simulink model "test_mdl_NI"  (R2018a)
settings: Solver=VariableStepAuto  StartTime=0.0  StopTime=10.0  RelTol=1e-3
(part 10 of 24)

== system test_mdl_NI/Subsystem/GWM/OTAPhysGWM_ECGtoSODCMC_Ox1B9114D8 ==
  in_port : Inport
  OTAPhysGWM_ECGtoSODCMC : Terminator
  bus_selector : BusSelector  OutputSignals=OTAPhysGWM_ECGtoSODCMC
  wires:
  in_port/1 -> bus_selector/1  "OTAPhysGWM_ECGtoSODCMC_Ox1B9114D8"
  bus_selector/1 -> OTAPhysGWM_ECGtoSODCMC/1  "<OTAPhysGWM_ECGtoSODCMC>"

== system test_mdl_NI/Subsystem/GWM/OTAPhysGWM_ECGtoSODCMD_Ox1B9118D8 ==
  in_port : Inport
  OTAPhysGWM_ECGtoSODCMD : Terminator
  bus_selector : BusSelector  OutputSignals=OTAPhysGWM_ECGtoSODCMD
  wires:
  in_port/1 -> bus_selector/1  "OTAPhysGWM_ECGtoSODCMD_Ox1B9118D8"
  bus_selector/1 -> OTAPhysGWM_ECGtoSODCMD/1  "<OTAPhysGWM_ECGtoSODCMD>"

== system test_mdl_NI/Subsystem/GWM/OTAPhysGWM_ECGtoSODL_Ox1B9188D8 ==
  in_port : Inport
  OTAPhysGWM_ECGtoSODL : Terminator
  bus_selector : BusSelector  OutputSignals=OTAPhysGWM_ECGtoSODL
  wires:
  in_port/1 -> bus_selector/1  "OTAPhysGWM_ECGtoSODL_Ox1B9188D8"
  bus_selector/1 -> OTAPhysGWM_ECGtoSODL/1  "<OTAPhysGWM_ECGtoSODL>"

== system test_mdl_NI/Subsystem/GWM/OTAPhysGWM_ECGtoSODR_Ox1B918CD8 ==
  in_port : Inport
  OTAPhysGWM_ECGtoSODR : Terminator
  bus_selector : BusSelector  OutputSignals=OTAPhysGWM_ECGtoSODR
  wires:
  in_port/1 -> bus_selector/1  "OTAPhysGWM_ECGtoSODR_Ox1B918CD8"
  bus_selector/1 -> OTAPhysGWM_ECGtoSODR/1  "<OTAPhysGWM_ECGtoSODR>"

== system test_mdl_NI/Subsystem/GWM/OffBrdChrg_Signals2_Ox27F ==
  in_port : Inport
  OfbChrgClearAll_B_Rq : Terminator
  OfbChrgGoTDelete_B_Rq : Terminator
  OfbChrgGoTElement_D_Rq : Terminator
  OfbChrgGoTExtHtr_D_Rq : Terminator
  OfbChrgGoTHr_T_Rq : Terminator
  OfbChrgGoTMnte_D_Rq : Terminator
  OfbChrgGoTOn_D_Rq : Terminator
  OfbChrgGoTPrcond_D_Rq : Terminator
  OfbChrgGoTTouch_D_Rq : Terminator
  OfbChrgGoTUpdate_B_Rq : Terminator
  OfbChrgPrflUpdate_B_Rq : Terminator
  bus_selector : BusSelector  OutputSignals=OfbChrgClearAll_B_Rq,OfbChrgGoTDelete_B_Rq,OfbChrgGoTElement_D_Rq,OfbChrgGoTExtHtr_D_Rq,OfbChrgGoTHr_T_Rq,OfbChrgGoTMnte_D_Rq,OfbChrgGoTOn_D_Rq,OfbChrgGoTPrcond_D_Rq,OfbChrgGoTTouch_D_Rq,OfbChrgGoTUpdate_B_Rq,OfbChrgPrflUpdate_B_Rq
  wires:
  in_port/1 -> bus_selector/1  "OffBrdChrg_Signals2_Ox27F"
  bus_selector/1 -> OfbChrgClearAll_B_Rq/1  "<OfbChrgClearAll_B_Rq>"
  bus_selector/2 -> OfbChrgGoTDelete_B_Rq/1  "<OfbChrgGoTDelete_B_Rq>"
  bus_selector/3 -> OfbChrgGoTElement_D_Rq/1  "<OfbChrgGoTElement_D_Rq>"
  bus_selector/4 -> OfbChrgGoTExtHtr_D_Rq/1  "<OfbChrgGoTExtHtr_D_Rq>"
  bus_selector/5 -> OfbChrgGoTHr_T_Rq/1  "<OfbChrgGoTHr_T_Rq>"
  bus_selector/6 -> OfbChrgGoTMnte_D_Rq/1  "<OfbChrgGoTMnte_D_Rq>"
  bus_selector/7 -> OfbChrgGoTOn_D_Rq/1  "<OfbChrgGoTOn_D_Rq>"
  bus_selector/8 -> OfbChrgGoTPrcond_D_Rq/1  "<OfbChrgGoTPrcond_D_Rq>"
  bus_selector/9 -> OfbChrgGoTTouch_D_Rq/1  "<OfbChrgGoTTouch_D_Rq>"
  bus_selector/10 -> OfbChrgGoTUpdate_B_Rq/1  "<OfbChrgGoTUpdate_B_Rq>"
  bus_selector/11 -> OfbChrgPrflUpdate_B_Rq/1  "<OfbChrgPrflUpdate_B_Rq>"

== system test_mdl_NI/Subsystem/GWM/OffBrdChrg_Signals_Ox212 ==
  in_port : Inport
  OfbChrgLocIdTrgt_No_Rq : Terminator
  OfbChrgLocIdUns_B_Rq : Terminator
  OfbChrgPrflWkdy_No_Rq : Terminator
  OfbChrgPrflWknd_No_Rq : Terminator
  OfbChrgSetDelete_B_Rq : Terminator
  OfbChrgSetNow_D_Rq : Terminator
  OfbChrgToPcWkdy_D_Actl : Terminator
  OfbChrgToPcWknd_D_Actl : Terminator
  bus_selector : BusSelector  OutputSignals=OfbChrgLocIdTrgt_No_Rq,OfbChrgLocIdUns_B_Rq,OfbChrgPrflWkdy_No_Rq,OfbChrgPrflWknd_No_Rq,OfbChrgSetDelete_B_Rq,OfbChrgSetNow_D_Rq,OfbChrgToPcWkdy_D_Actl,OfbChrgToPcWknd_D_Actl
  wires:
  in_port/1 -> bus_selector/1  "OffBrdChrg_Signals_Ox212"
  bus_selector/1 -> OfbChrgLocIdTrgt_No_Rq/1  "<OfbChrgLocIdTrgt_No_Rq>"
  bus_selector/2 -> OfbChrgLocIdUns_B_Rq/1  "<OfbChrgLocIdUns_B_Rq>"
  bus_selector/3 -> OfbChrgPrflWkdy_No_Rq/1  "<OfbChrgPrflWkdy_No_Rq>"
  bus_selector/4 -> OfbChrgPrflWknd_No_Rq/1  "<OfbChrgPrflWknd_No_Rq>"
  bus_selector/5 -> OfbChrgSetDelete_B_Rq/1  "<OfbChrgSetDelete_B_Rq>"
  bus_selector/6 -> OfbChrgSetNow_D_Rq/1  "<OfbChrgSetNow_D_Rq>"
  bus_selector/7 -> OfbChrgToPcWkdy_D_Actl/1  "<OfbChrgToPcWkdy_D_Actl>"
  bus_selector/8 -> OfbChrgToPcWknd_D_Actl/1  "<OfbChrgToPcWknd_D_Actl>"

== system test_mdl_NI/Subsystem/GWM/PARSEDFuncGWM_ECG_FD1_Ox1BAFFCD8 ==
  in_port : Inport
  PARSEDFuncGWM_ECG : Terminator
  bus_selector : BusSelector  OutputSignals=PARSEDFuncGWM_ECG
  wires:
  in_port/1 -> bus_selector/1  "PARSEDFuncGWM_ECG_FD1_Ox1BAFFCD8"
  bus_selector/1 -> PARSEDFuncGWM_ECG/1  "<PARSEDFuncGWM_ECG>"

== system test_mdl_NI/Subsystem/GWM/PARSEDPhysGWM_ECGtoABS_Ox1BA0A0D8 ==
  in_port : Inport
  PARSEDPhysGWM_ECGtoABS : Terminator
  bus_selector : BusSelector  OutputSignals=PARSEDPhysGWM_ECGtoABS
  wires:
  in_port/1 -> bus_selector/1  "PARSEDPhysGWM_ECGtoABS_Ox1BA0A0D8"
  bus_selector/1 -> PARSEDPhysGWM_ECGtoABS/1  "<PARSEDPhysGWM_ECGtoABS>"

== system test_mdl_NI/Subsystem/GWM/PARSEDPhysGWM_ECGtoCCM_Ox1BA054D8 ==
  in_port : Inport
  PARSEDPhysGWM_ECGtoCCM : Terminator
  bus_selector : BusSelector  OutputSignals=PARSEDPhysGWM_ECGtoCCM
  wires:
  in_port/1 -> bus_selector/1  "PARSEDPhysGWM_ECGtoCCM_Ox1BA054D8"
  bus_selector/1 -> PARSEDPhysGWM_ECGtoCCM/1  "<PARSEDPhysGWM_ECGtoCCM>"

== system test_mdl_NI/Subsystem/GWM/PARSEDPhysGWM_ECGtoIPMA_Ox1BA084D8 ==
  in_port : Inport
  PARSEDPhysGWM_ECGtoIPMA : Terminator
  bus_selector : BusSelector  OutputSignals=PARSEDPhysGWM_ECGtoIPMA
  wires:
  in_port/1 -> bus_selector/1  "PARSEDPhysGWM_ECGtoIPMA_Ox1BA084D8"
  bus_selector/1 -> PARSEDPhysGWM_ECGtoIPMA/1  "<PARSEDPhysGWM_ECGtoIPMA>"

== system test_mdl_NI/Subsystem/GWM/PARSEDPhysGWM_ECGtoPCM_Ox1BA040D8 ==
  in_port : Inport
  PARSEDPhysGWM_ECGtoPCM : Terminator
  bus_selector : BusSelector  OutputSignals=PARSEDPhysGWM_ECGtoPCM
  wires:
  in_port/1 -> bus_selector/1  "PARSEDPhysGWM_ECGtoPCM_Ox1BA040D8"
  bus_selector/1 -> PARSEDPhysGWM_ECGtoPCM/1  "<PARSEDPhysGWM_ECGtoPCM>"

== system test_mdl_NI/Subsystem/GWM/PARSEDPhysGWM_ECGtoSODCMC_Ox1BA114D8 ==
  in_port : Inport
  PARSEDPhysGWM_ECGtoSODCMC : Terminator
  bus_selector : BusSelector  OutputSignals=PARSEDPhysGWM_ECGtoSODCMC
  wires:
  in_port/1 -> bus_selector/1  "PARSEDPhysGWM_ECGtoSODCMC_Ox1BA114D8"
  bus_selector/1 -> PARSEDPhysGWM_ECGtoSODCMC/1  "<PARSEDPhysGWM_ECGtoSODCMC>"

== system test_mdl_NI/Subsystem/GWM/PARSEDPhysGWM_ECGtoSODCMD_Ox1BA118D8 ==
  in_port : Inport
  PARSEDPhysGWM_ECGtoSODCMD : Terminator
  bus_selector : BusSelector  OutputSignals=PARSEDPhysGWM_ECGtoSODCMD
  wires:
  in_port/1 -> bus_selector/1  "PARSEDPhysGWM_ECGtoSODCMD_Ox1BA118D8"
  bus_selector/1 -> PARSEDPhysGWM_ECGtoSODCMD/1  "<PARSEDPhysGWM_ECGtoSODCMD>"

== system test_mdl_NI/Subsystem/GWM/PARSEDPhysGWM_ECGtoSODL_Ox1BA188D8 ==
  in_port : Inport
  PARSEDPhysGWM_ECGtoSODL : Terminator
  bus_selector : BusSelector  OutputSignals=PARSEDPhysGWM_ECGtoSODL
  wires:
  in_port/1 -> bus_selector/1  "PARSEDPhysGWM_ECGtoSODL_Ox1BA188D8"
  bus_selector/1 -> PARSEDPhysGWM_ECGtoSODL/1  "<PARSEDPhysGWM_ECGtoSODL>"

== system test_mdl_NI/Subsystem/GWM/PARSEDPhysGWM_ECGtoSODR_Ox1BA18CD8 ==
  in_port : Inport
  PARSEDPhysGWM_ECGtoSODR : Terminator
  bus_selector : BusSelector  OutputSignals=PARSEDPhysGWM_ECGtoSODR
  wires:
  in_port/1 -> bus_selector/1  "PARSEDPhysGWM_ECGtoSODR_Ox1BA18CD8"
  bus_selector/1 -> PARSEDPhysGWM_ECGtoSODR/1  "<PARSEDPhysGWM_ECGtoSODR>"

== system test_mdl_NI/Subsystem/GWM/PARSEDPhysGWMtoSOBDMC_FD1_Ox1BA044D8 ==
  in_port : Inport
  PARSEDPhysGWM_ECGtoHPCM : Terminator
  bus_selector : BusSelector  OutputSignals=PARSEDPhysGWM_ECGtoHPCM
  wires:
  in_port/1 -> bus_selector/1  "PARSEDPhysGWMtoSOBDMC_FD1_Ox1BA044D8"
  bus_selector/1 -> PARSEDPhysGWM_ECGtoHPCM/1  "<PARSEDPhysGWM_ECGtoHPCM>"

== system test_mdl_NI/Subsystem/GWM/PARSEDPushFcGWM_ECGtoABS_Ox1BB0A0D8 ==
  in_port : Inport
  PARSEDPhysGWM_ECG2toABS : Terminator
  bus_selector : BusSelector  OutputSignals=PARSEDPhysGWM_ECG2toABS
  wires:
  in_port/1 -> bus_selector/1  "PARSEDPushFcGWM_ECGtoABS_Ox1BB0A0D8"
  bus_selector/1 -> PARSEDPhysGWM_ECG2toABS/1  "<PARSEDPhysGWM_ECG2toABS>"

== system test_mdl_NI/Subsystem/GWM/PARSEDPushFcGWM_ECGtoPCM_Ox1BB040D8 ==
  in_port : Inport
  PARSEDPhysGWM_ECG2toPCM : Terminator
  bus_selector : BusSelector  OutputSignals=PARSEDPhysGWM_ECG2toPCM
  wires:
  in_port/1 -> bus_selector/1  "PARSEDPushFcGWM_ECGtoPCM_Ox1BB040D8"
  bus_selector/1 -> PARSEDPhysGWM_ECG2toPCM/1  "<PARSEDPhysGWM_ECG2toPCM>"

== system test_mdl_NI/Subsystem/GWM/PHEV_Battery_Data1_FD1_Ox2E4 ==
  in_port : Inport
  BattAuxCnnct_B_Cmd : Terminator
  bus_selector : BusSelector  OutputSignals=BattAuxCnnct_B_Cmd
  wires:
  in_port/1 -> bus_selector/1  "PHEV_Battery_Data1_FD1_Ox2E4"
  bus_selector/1 -> BattAuxCnnct_B_Cmd/1  "<BattAuxCnnct_B_Cmd>"

== system test_mdl_NI/Subsystem/GWM/ParkAid_Aud_Warn_CmdM_FD1_Ox30A ==
  in_port : Inport
  Cta_D_Rq : Terminator
  PrkAidAcsyFront_D_RqDrv : Terminator
  PrkAidAcsyRear_D_RqDrv : Terminator
  PrkAidFront_D_RqDrv : Terminator
  PrkAidRear_D_RqDrv : Terminator
  Sod_D_Rq : Terminator
  SteEffort_D_Rq : Terminator
  bus_selector : BusSelector  OutputSignals=Cta_D_Rq,PrkAidAcsyFront_D_RqDrv,PrkAidAcsyRear_D_RqDrv,PrkAidFront_D_RqDrv,PrkAidRear_D_RqDrv,Sod_D_Rq,SteEffort_D_Rq
  wires:
  in_port/1 -> bus_selector/1  "ParkAid_Aud_Warn_CmdM_FD1_Ox30A"
  bus_selector/1 -> Cta_D_Rq/1  "<Cta_D_Rq>"
  bus_selector/2 -> PrkAidAcsyFront_D_RqDrv/1  "<PrkAidAcsyFront_D_RqDrv>"
  bus_selector/3 -> PrkAidAcsyRear_D_RqDrv/1  "<PrkAidAcsyRear_D_RqDrv>"
  bus_selector/4 -> PrkAidFront_D_RqDrv/1  "<PrkAidFront_D_RqDrv>"
  bus_selector/5 -> PrkAidRear_D_RqDrv/1  "<PrkAidRear_D_RqDrv>"
  bus_selector/6 -> Sod_D_Rq/1  "<Sod_D_Rq>"
  bus_selector/7 -> SteEffort_D_Rq/1  "<SteEffort_D_Rq>"

== system test_mdl_NI/Subsystem/GWM/Pass_Dr_Stat_FD1_Ox333 ==
  in_port : Inport
  BLISLEDStatPassSide : Terminator
  ChildLckFdbckRp_B_Stat : Terminator
  Memory_1_SwPsngr_Stat : Terminator
  Memory_2_SwPsngr_Stat : Terminator
  Memory_3_SwPsngr_Stat : Terminator
  Pasngr_Lock_Sw_Cnt : Terminator
  Pasngr_Lock_Sw_Stat : Terminator
  RollCode_No_ActlPdm : Terminator
  WndwPsngrSide_D_Stat : Terminator
  bus_selector : BusSelector  OutputSignals=BLISLEDStatPassSide,ChildLckFdbckRp_B_Stat,Memory_1_SwPsngr_Stat,Memory_2_SwPsngr_Stat,Memory_3_SwPsngr_Stat,Pasngr_Lock_Sw_Cnt,Pasngr_Lock_Sw_Stat,RollCode_No_ActlPdm,WndwPsngrSide_D_Stat
  wires:
  in_port/1 -> bus_selector/1  "Pass_Dr_Stat_FD1_Ox333"
  bus_selector/1 -> BLISLEDStatPassSide/1  "<BLISLEDStatPassSide>"
  bus_selector/2 -> ChildLckFdbckRp_B_Stat/1  "<ChildLckFdbckRp_B_Stat>"
  bus_selector/3 -> Memory_1_SwPsngr_Stat/1  "<Memory_1_SwPsngr_Stat>"
  bus_selector/4 -> Memory_2_SwPsngr_Stat/1  "<Memory_2_SwPsngr_Stat>"
  bus_selector/5 -> Memory_3_SwPsngr_Stat/1  "<Memory_3_SwPsngr_Stat>"
  bus_selector/6 -> Pasngr_Lock_Sw_Cnt/1  "<Pasngr_Lock_Sw_Cnt>"
  bus_selector/7 -> Pasngr_Lock_Sw_Stat/1  "<Pasngr_Lock_Sw_Stat>"
  bus_selector/8 -> RollCode_No_ActlPdm/1  "<RollCode_No_ActlPdm>"
  bus_selector/9 -> WndwPsngrSide_D_Stat/1  "<WndwPsngrSide_D_Stat>"

== system test_mdl_NI/Subsystem/GWM/Personality_APIM_Data_FD1_Ox3E2 ==
  in_port : Inport
  CtrStkDsplyOp_D_Rq : Terminator
  CtrStkFeatConfigActl : Terminator
  CtrStkFeatNoActl : Terminator
  CtrStkPersIndex_D_Actl : Terminator
  Pers1OptIn_B_Stats : Terminator
  Pers2OptIn_B_Stats : Terminator
  Pers3OptIn_B_Stats : Terminator
  Pers4OptIn_B_Stats : Terminator
  PersStore_D_Rq : Terminator
  bus_selector : BusSelector  OutputSignals=CtrStkDsplyOp_D_Rq,CtrStkFeatConfigActl,CtrStkFeatNoActl,CtrStkPersIndex_D_Actl,Pers1OptIn_B_Stats,Pers2OptIn_B_Stats,Pers3OptIn_B_Stats,Pers4OptIn_B_Stats,PersStore_D_Rq
  wires:
  in_port/1 -> bus_selector/1  "Personality_APIM_Data_FD1_Ox3E2"
  bus_selector/1 -> CtrStkDsplyOp_D_Rq/1  "<CtrStkDsplyOp_D_Rq>"
  bus_selector/2 -> CtrStkFeatConfigActl/1  "<CtrStkFeatConfigActl>"
  bus_selector/3 -> CtrStkFeatNoActl/1  "<CtrStkFeatNoActl>"
  bus_selector/4 -> CtrStkPersIndex_D_Actl/1  "<CtrStkPersIndex_D_Actl>"
  bus_selector/5 -> Pers1OptIn_B_Stats/1  "<Pers1OptIn_B_Stats>"
  bus_selector/6 -> Pers2OptIn_B_Stats/1  "<Pers2OptIn_B_Stats>"
  bus_selector/7 -> Pers3OptIn_B_Stats/1  "<Pers3OptIn_B_Stats>"
  bus_selector/8 -> Pers4OptIn_B_Stats/1  "<Pers4OptIn_B_Stats>"
  bus_selector/9 -> PersStore_D_Rq/1  "<PersStore_D_Rq>"

== system test_mdl_NI/Subsystem/GWM/Personality_BCM2_Data_FD1_Ox3EB ==
  in_port : Inport
  AssocConfirm_D_Actl : Terminator
  EmPrflKeyAssoc_D_Stat : Terminator
  EmPrflNo_D_Stat : Terminator
  Pers1Key_D_Stat : Terminator
  Pers2Key_D_Stat : Terminator
  Pers3Key_D_Stat : Terminator
  Pers4Key_D_Stat : Terminator
  PersConflict_D_Actl : Terminator
  PersNoPos_D_Actl : Terminator
  PersNo_D_Actl : Terminator
  PersRecallSrc_D_Actl : Terminator
  PersSetupAccessCtrl : Terminator
  PersSetupRestr_D_Actl : Terminator
  PersSetup_No_Actl : Terminator
  RecallEvent_No_Cnt : Terminator
  VehKeyActv_D_Stat : Terminator
  bus_selector : BusSelector  OutputSignals=AssocConfirm_D_Actl,EmPrflKeyAssoc_D_Stat,EmPrflNo_D_Stat,Pers1Key_D_Stat,Pers2Key_D_Stat,Pers3Key_D_Stat,Pers4Key_D_Stat,PersConflict_D_Actl,PersNoPos_D_Actl,PersNo_D_Actl,PersRecallSrc_D_Actl,PersSetupAccessCtrl,PersSetupRestr_D_Actl,PersSetup_No_Actl,RecallEvent_No_Cnt,VehKeyActv_D_Stat
  wires:
  in_port/1 -> bus_selector/1  "Personality_BCM2_Data_FD1_Ox3EB"
  bus_selector/1 -> AssocConfirm_D_Actl/1  "<AssocConfirm_D_Actl>"
  bus_selector/2 -> EmPrflKeyAssoc_D_Stat/1  "<EmPrflKeyAssoc_D_Stat>"
  bus_selector/3 -> EmPrflNo_D_Stat/1  "<EmPrflNo_D_Stat>"
  bus_selector/4 -> Pers1Key_D_Stat/1  "<Pers1Key_D_Stat>"
  bus_selector/5 -> Pers2Key_D_Stat/1  "<Pers2Key_D_Stat>"
  bus_selector/6 -> Pers3Key_D_Stat/1  "<Pers3Key_D_Stat>"
  bus_selector/7 -> Pers4Key_D_Stat/1  "<Pers4Key_D_Stat>"
  bus_selector/8 -> PersConflict_D_Actl/1  "<PersConflict_D_Actl>"
  bus_selector/9 -> PersNoPos_D_Actl/1  "<PersNoPos_D_Actl>"
  bus_selector/10 -> PersNo_D_Actl/1  "<PersNo_D_Actl>"
  bus_selector/11 -> PersRecallSrc_D_Actl/1  "<PersRecallSrc_D_Actl>"
  bus_selector/12 -> PersSetupAccessCtrl/1  "<PersSetupAccessCtrl>"
  bus_selector/13 -> PersSetupRestr_D_Actl/1  "<PersSetupRestr_D_Actl>"
  bus_selector/14 -> PersSetup_No_Actl/1  "<PersSetup_No_Actl>"
  bus_selector/15 -> RecallEvent_No_Cnt/1  "<RecallEvent_No_Cnt>"
  bus_selector/16 -> VehKeyActv_D_Stat/1  "<VehKeyActv_D_Stat>"

== system test_mdl_NI/Subsystem/GWM/Personality_Data_FD1_Ox3E0 ==
  in_port : Inport
  MsgCntrDsplyOp_D_Rq : Terminator
  MsgCntrFeatConfigRq : Terminator
  MsgCntrFeatNoRq : Terminator
  MsgCntrPersIndex_D_Rq : Terminator
  bus_selector : BusSelector  OutputSignals=MsgCntrDsplyOp_D_Rq,MsgCntrFeatConfigRq,MsgCntrFeatNoRq,MsgCntrPersIndex_D_Rq
  wires:
  in_port/1 -> bus_selector/1  "Personality_Data_FD1_Ox3E0"
  bus_selector/1 -> MsgCntrDsplyOp_D_Rq/1  "<MsgCntrDsplyOp_D_Rq>"
  bus_selector/2 -> MsgCntrFeatConfigRq/1  "<MsgCntrFeatConfigRq>"
  bus_selector/3 -> MsgCntrFeatNoRq/1  "<MsgCntrFeatNoRq>"
  bus_selector/4 -> MsgCntrPersIndex_D_Rq/1  "<MsgCntrPersIndex_D_Rq>"

== system test_mdl_NI/Subsystem/GWM/PowerDistData_2_FD1_Ox36A ==
  in_port : Inport
  AirCondCluBatt_D_Falt : Terminator
  AirCondCluGnd_D_Falt : Terminator
  AirCondCluLife_D_Falt : Terminator
  AirCondCluOpen_D_Falt : Terminator
  AirCondClu_D_Stat : Terminator
  BattChlrLifeLim_D_Falt : Terminator
  BattChlrOpnCirct_D_Falt : Terminator
  BattChlrShrtBatt_D_Falt : Terminator
  BattChlrShrtGrnd_D_Falt : Terminator
  BattTracLifeLim_D_Falt : Terminator
  BattTracLow_D_Falt : Terminator
  BattTracOpnCirct_D_Falt : Terminator
  BattTracShrtBatt_D_Falt : Terminator
  BattTracShrtGrnd_D_Falt : Terminator
  bus_selector : BusSelector  OutputSignals=AirCondCluBatt_D_Falt,AirCondCluGnd_D_Falt,AirCondCluLife_D_Falt,AirCondCluOpen_D_Falt,AirCondClu_D_Stat,BattChlrLifeLim_D_Falt,BattChlrOpnCirct_D_Falt,BattChlrShrtBatt_D_Falt,BattChlrShrtGrnd_D_Falt,BattTracLifeLim_D_Falt,BattTracLow_D_Falt,BattTracOpnCirct_D_Falt,BattTracShrtBatt_D_Falt,BattTracShrtGrnd_D_Falt
  wires:
  in_port/1 -> bus_selector/1  "PowerDistData_2_FD1_Ox36A"
  bus_selector/1 -> AirCondCluBatt_D_Falt/1  "<AirCondCluBatt_D_Falt>"
  bus_selector/2 -> AirCondCluGnd_D_Falt/1  "<AirCondCluGnd_D_Falt>"
  bus_selector/3 -> AirCondCluLife_D_Falt/1  "<AirCondCluLife_D_Falt>"
  bus_selector/4 -> AirCondCluOpen_D_Falt/1  "<AirCondCluOpen_D_Falt>"
  bus_selector/5 -> AirCondClu_D_Stat/1  "<AirCondClu_D_Stat>"
  bus_selector/6 -> BattChlrLifeLim_D_Falt/1  "<BattChlrLifeLim_D_Falt>"
  bus_selector/7 -> BattChlrOpnCirct_D_Falt/1  "<BattChlrOpnCirct_D_Falt>"
  bus_selector/8 -> BattChlrShrtBatt_D_Falt/1  "<BattChlrShrtBatt_D_Falt>"
  bus_selector/9 -> BattChlrShrtGrnd_D_Falt/1  "<BattChlrShrtGrnd_D_Falt>"
  bus_selector/10 -> BattTracLifeLim_D_Falt/1  "<BattTracLifeLim_D_Falt>"
  bus_selector/11 -> BattTracLow_D_Falt/1  "<BattTracLow_D_Falt>"
  bus_selector/12 -> BattTracOpnCirct_D_Falt/1  "<BattTracOpnCirct_D_Falt>"
  bus_selector/13 -> BattTracShrtBatt_D_Falt/1  "<BattTracShrtBatt_D_Falt>"
  bus_selector/14 -> BattTracShrtGrnd_D_Falt/1  "<BattTracShrtGrnd_D_Falt>"

== system test_mdl_NI/Subsystem/GWM/PowerDist_Data1_FD1_Ox390 ==
  in_port : Inport
  BattChlrSov_D_Stat : Terminator
  BattTracClntVlv_D_Stat : Terminator
  CabnEvapSovFront_D_Stat : Terminator
  bus_selector : BusSelector  OutputSignals=BattChlrSov_D_Stat,BattTracClntVlv_D_Stat,CabnEvapSovFront_D_Stat
  wires:
  in_port/1 -> bus_selector/1  "PowerDist_Data1_FD1_Ox390"
  bus_selector/1 -> BattChlrSov_D_Stat/1  "<BattChlrSov_D_Stat>"
  bus_selector/2 -> BattTracClntVlv_D_Stat/1  "<BattTracClntVlv_D_Stat>"
  bus_selector/3 -> CabnEvapSovFront_D_Stat/1  "<CabnEvapSovFront_D_Stat>"

== system test_mdl_NI/Subsystem/GWM/Power_Liftgate_Stat_FD1_Ox313 ==
  in_port : Inport
  DrLckCnt_No_ActlTgate : Terminator
  DrTGate_D_Rq : Terminator
  DrTgateChime2_D_Rq : Terminator
  Power_Liftgate_Mode_Stt : Terminator
  PwLftgtIntSw_B_Stat : Terminator
  bus_selector : BusSelector  OutputSignals=DrLckCnt_No_ActlTgate,DrTGate_D_Rq,DrTgateChime2_D_Rq,Power_Liftgate_Mode_Stt,PwLftgtIntSw_B_Stat
  wires:
  in_port/1 -> bus_selector/1  "Power_Liftgate_Stat_FD1_Ox313"
  bus_selector/1 -> DrLckCnt_No_ActlTgate/1  "<DrLckCnt_No_ActlTgate>"
  bus_selector/2 -> DrTGate_D_Rq/1  "<DrTGate_D_Rq>"
  bus_selector/3 -> DrTgateChime2_D_Rq/1  "<DrTgateChime2_D_Rq>"
  bus_selector/4 -> Power_Liftgate_Mode_Stt/1  "<Power_Liftgate_Mode_Stt>"
  bus_selector/5 -> PwLftgtIntSw_B_Stat/1  "<PwLftgtIntSw_B_Stat>"

== system test_mdl_NI/Subsystem/GWM/RCMSerialNumber_FD1_Ox454 ==
  in_port : Inport
  RCMSerialNoByte{1..8} (8 alike) : Terminator
  bus_selector : BusSelector  OutputSignals=RCMSerialNoByte1,RCMSerialNoByte2,RCMSerialNoByte3,RCMSerialNoByte4,RCMSerialNoByte5,RCMSerialNoByte6,RCMSerialNoByte7,RCMSerialNoByte8
  wires:
  in_port/1 -> bus_selector/1  "RCMSerialNumber_FD1_Ox454"
  bus_selector/1 -> RCMSerialNoByte1/1  "<RCMSerialNoByte1>"
  bus_selector/2 -> RCMSerialNoByte2/1  "<RCMSerialNoByte2>"
  bus_selector/3 -> RCMSerialNoByte3/1  "<RCMSerialNoByte3>"
  bus_selector/4 -> RCMSerialNoByte4/1  "<RCMSerialNoByte4>"
  bus_selector/5 -> RCMSerialNoByte5/1  "<RCMSerialNoByte5>"
  bus_selector/6 -> RCMSerialNoByte6/1  "<RCMSerialNoByte6>"
  bus_selector/7 -> RCMSerialNoByte7/1  "<RCMSerialNoByte7>"
  bus_selector/8 -> RCMSerialNoByte8/1  "<RCMSerialNoByte8>"

== system test_mdl_NI/Subsystem/GWM/RCMStatusMessage2_FD1_Ox4C ==
  in_port : Inport
  EDRTriggerEvntSync : Terminator
  FirstRowBuckleDriver : Terminator
  FirstRowBuckleMid : Terminator
  FirstRowBucklePsngr : Terminator
  PassRstrnInd_Req : Terminator
  PsngrFrntDetct_D_Actl : Terminator
  RILReq : Terminator
  RstrnImpactEvntStatus : Terminator
  SecondRowBuckleDriver : Terminator
  SecondRowBuckleMid : Terminator
  SecondRowBucklePsngr : Terminator
  bus_selector : BusSelector  OutputSignals=EDRTriggerEvntSync,FirstRowBuckleDriver,FirstRowBuckleMid,FirstRowBucklePsngr,PassRstrnInd_Req,PsngrFrntDetct_D_Actl,RILReq,RstrnImpactEvntStatus,SecondRowBuckleDriver,SecondRowBuckleMid,SecondRowBucklePsngr
  wires:
  in_port/1 -> bus_selector/1  "RCMStatusMessage2_FD1_Ox4C"
  bus_selector/1 -> EDRTriggerEvntSync/1  "<EDRTriggerEvntSync>"
  bus_selector/2 -> FirstRowBuckleDriver/1  "<FirstRowBuckleDriver>"
  bus_selector/3 -> FirstRowBuckleMid/1  "<FirstRowBuckleMid>"
  bus_selector/4 -> FirstRowBucklePsngr/1  "<FirstRowBucklePsngr>"
  bus_selector/5 -> PassRstrnInd_Req/1  "<PassRstrnInd_Req>"
  bus_selector/6 -> PsngrFrntDetct_D_Actl/1  "<PsngrFrntDetct_D_Actl>"
  bus_selector/7 -> RILReq/1  "<RILReq>"
  bus_selector/8 -> RstrnImpactEvntStatus/1  "<RstrnImpactEvntStatus>"
  bus_selector/9 -> SecondRowBuckleDriver/1  "<SecondRowBuckleDriver>"
  bus_selector/10 -> SecondRowBuckleMid/1  "<SecondRowBuckleMid>"
  bus_selector/11 -> SecondRowBucklePsngr/1  "<SecondRowBucklePsngr>"

== system test_mdl_NI/Subsystem/GWM/SmartChargingData_ECG_1_Ox306 ==
  in_port : Inport
  ScLocDelete_B_RqCld : Terminator
  ScLocId_No_RqCld : Terminator
  ScLocLattDeg_An_RqCld : Terminator
  ScLocLattFrct_An_RqCld : Terminator
  ScLocLattPostv_B_RqCld : Terminator
  ScLocLongDeg_An_RqCld : Terminator
  ScLocLongFrct_An_RqCld : Terminator
  ScLocLongPostv_B_RqCld : Terminator
  bus_selector : BusSelector  OutputSignals=ScLocDelete_B_RqCld,ScLocId_No_RqCld,ScLocLattDeg_An_RqCld,ScLocLattFrct_An_RqCld,ScLocLattPostv_B_RqCld,ScLocLongDeg_An_RqCld,ScLocLongFrct_An_RqCld,ScLocLongPostv_B_RqCld
  wires:
  in_port/1 -> bus_selector/1  "SmartChargingData_ECG_1_Ox306"
  bus_selector/1 -> ScLocDelete_B_RqCld/1  "<ScLocDelete_B_RqCld>"
  bus_selector/2 -> ScLocId_No_RqCld/1  "<ScLocId_No_RqCld>"
  bus_selector/3 -> ScLocLattDeg_An_RqCld/1  "<ScLocLattDeg_An_RqCld>"
  bus_selector/4 -> ScLocLattFrct_An_RqCld/1  "<ScLocLattFrct_An_RqCld>"
  bus_selector/5 -> ScLocLattPostv_B_RqCld/1  "<ScLocLattPostv_B_RqCld>"
  bus_selector/6 -> ScLocLongDeg_An_RqCld/1  "<ScLocLongDeg_An_RqCld>"
  bus_selector/7 -> ScLocLongFrct_An_RqCld/1  "<ScLocLongFrct_An_RqCld>"
  bus_selector/8 -> ScLocLongPostv_B_RqCld/1  "<ScLocLongPostv_B_RqCld>"

== system test_mdl_NI/Subsystem/GWM/SmartChargingData_ECG_2_Ox307 ==
  in_port : Inport
  ScChrgDurSet_D_RqCld : Terminator
  ScChrgDur_T_RqCld : Terminator
  ScChrgPrfl_No_RqCld : Terminator
  ScChrgToPc_Pc_RqCld : Terminator
  ScDayOfWeekId_D_RqCld : Terminator
  ScLocRdius_L_RqCld : Terminator
  ScLocSetId_No_RqCld : Terminator
  bus_selector : BusSelector  OutputSignals=ScChrgDurSet_D_RqCld,ScChrgDur_T_RqCld,ScChrgPrfl_No_RqCld,ScChrgToPc_Pc_RqCld,ScDayOfWeekId_D_RqCld,ScLocRdius_L_RqCld,ScLocSetId_No_RqCld
  wires:
  in_port/1 -> bus_selector/1  "SmartChargingData_ECG_2_Ox307"
  bus_selector/1 -> ScChrgDurSet_D_RqCld/1  "<ScChrgDurSet_D_RqCld>"
  bus_selector/2 -> ScChrgDur_T_RqCld/1  "<ScChrgDur_T_RqCld>"
  bus_selector/3 -> ScChrgPrfl_No_RqCld/1  "<ScChrgPrfl_No_RqCld>"
  bus_selector/4 -> ScChrgToPc_Pc_RqCld/1  "<ScChrgToPc_Pc_RqCld>"
  bus_selector/5 -> ScDayOfWeekId_D_RqCld/1  "<ScDayOfWeekId_D_RqCld>"
  bus_selector/6 -> ScLocRdius_L_RqCld/1  "<ScLocRdius_L_RqCld>"
  bus_selector/7 -> ScLocSetId_No_RqCld/1  "<ScLocSetId_No_RqCld>"

== system test_mdl_NI/Subsystem/GWM/SmartChargingData_ECG_3_Ox308 ==
  in_port : Inport
  AirAmb_Te_ActlCld : Terminator
  ChrgToPcEdit_Pc_RqCld : Terminator
  GoTEditHr_T_RqCld : Terminator
  GoTEditMnte_T_RqCld : Terminator
  PrcondEdit_D_RqCld : Terminator
  ScChrgrPwMax_Pw_RqCld : Terminator
  ScEnbl_D_RqCld : Terminator
  ScFreshDataEnbl_B_Rq : Terminator
  ScLocPwId_No_RqCld : Terminator
  ScMnSoc_Pc_RqCld : Terminator
  bus_selector : BusSelector  OutputSignals=AirAmb_Te_ActlCld,ChrgToPcEdit_Pc_RqCld,GoTEditHr_T_RqCld,GoTEditMnte_T_RqCld,PrcondEdit_D_RqCld,ScChrgrPwMax_Pw_RqCld,ScEnbl_D_RqCld,ScFreshDataEnbl_B_Rq,ScLocPwId_No_RqCld,ScMnSoc_Pc_RqCld
  wires:
  in_port/1 -> bus_selector/1  "SmartChargingData_ECG_3_Ox308"
  bus_selector/1 -> AirAmb_Te_ActlCld/1  "<AirAmb_Te_ActlCld>"
  bus_selector/2 -> ChrgToPcEdit_Pc_RqCld/1  "<ChrgToPcEdit_Pc_RqCld>"
  bus_selector/3 -> GoTEditHr_T_RqCld/1  "<GoTEditHr_T_RqCld>"
  bus_selector/4 -> GoTEditMnte_T_RqCld/1  "<GoTEditMnte_T_RqCld>"
  bus_selector/5 -> PrcondEdit_D_RqCld/1  "<PrcondEdit_D_RqCld>"
  bus_selector/6 -> ScChrgrPwMax_Pw_RqCld/1  "<ScChrgrPwMax_Pw_RqCld>"
  bus_selector/7 -> ScEnbl_D_RqCld/1  "<ScEnbl_D_RqCld>"
  bus_selector/8 -> ScFreshDataEnbl_B_Rq/1  "<ScFreshDataEnbl_B_Rq>"
  bus_selector/9 -> ScLocPwId_No_RqCld/1  "<ScLocPwId_No_RqCld>"
  bus_selector/10 -> ScMnSoc_Pc_RqCld/1  "<ScMnSoc_Pc_RqCld>"

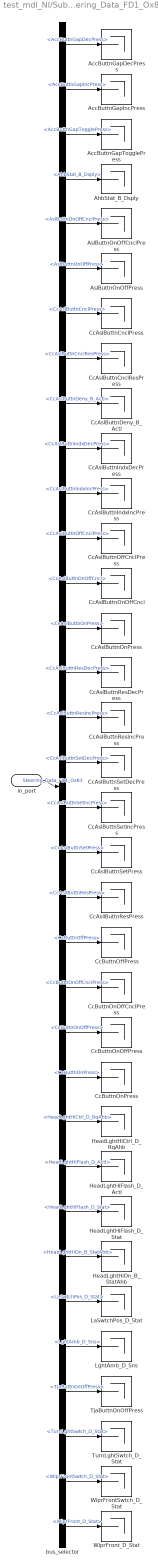
== system test_mdl_NI/Subsystem/GWM/Steering_Data_FD1_Ox83 ==
  in_port : Inport
  AccButtnGapDecPress : Terminator
  AccButtnGapIncPress : Terminator
  AccButtnGapTogglePress : Terminator
  AhbStat_B_Dsply : Terminator
  AslButtnOnOffCnclPress : Terminator
  AslButtnOnOffPress : Terminator
  CcAslButtnCnclPress : Terminator
  CcAslButtnCnclResPress : Terminator
  CcAslButtnDeny_B_Actl : Terminator
  CcAslButtnIndxDecPress : Terminator
  CcAslButtnIndxIncPress : Terminator
  CcAslButtnOffCnclPress : Terminator
  CcAslButtnOnOffCncl : Terminator
  CcAslButtnOnPress : Terminator
  CcAslButtnResDecPress : Terminator
  CcAslButtnResIncPress : Terminator
  CcAslButtnSetDecPress : Terminator
  CcAslButtnSetIncPress : Terminator
  CcAslButtnSetPress : Terminator
  CcAsllButtnResPress : Terminator
  CcButtnOffPress : Terminator
  CcButtnOnOffCnclPress : Terminator
  CcButtnOnOffPress : Terminator
  CcButtnOnPress : Terminator
  HeadLghtHiCtrl_D_RqAhb : Terminator
  HeadLghtHiFlash_D_Actl : Terminator
  HeadLghtHiFlash_D_Stat : Terminator
  HeadLghtHiOn_B_StatAhb : Terminator
  LaSwtchPos_D_Stat : Terminator
  LghtAmb_D_Sns : Terminator
  TjaButtnOnOffPress : Terminator
  TurnLghtSwtch_D_Stat : Terminator
  WiprFrontSwtch_D_Stat : Terminator
  WiprFront_D_Stat : Terminator
  bus_selector : BusSelector  OutputSignals=AccButtnGapDecPress,AccButtnGapIncPress,AccButtnGapTogglePress,AhbStat_B_Dsply,AslButtnOnOffCnclPress,AslButtnOnOffPress,CcAslButtnCnclPress,CcAslButtnCnclResPress,CcAslButtnDeny_B_Actl,CcAslButtnIndxDecPress,CcAslButtnIndxIncPress,CcAslButtnOffCnclPress,CcAslButtnOnOffCncl,CcAslButtnOnPress,CcAslButtnResDecPress,CcAslButtnResIncPress,CcAslButtnSetDecPress,CcAslButtnSetIncPress,CcAslButtnSetPress,CcAsllButtnResPress,CcButtnOffPress,CcButtnOnOffCnclPress,CcButtnOnOffPress,CcButtnOnPress,HeadLghtHiCtrl_D_RqAhb,HeadLghtHiFlash_D_Actl,HeadLghtHiFlash_D_Stat,HeadLghtHiOn_B_StatAhb,LaSwtchPos_D_Stat,LghtAmb_D_Sns,TjaButtnOnOffPress,TurnLghtSwtch_D_Stat,WiprFrontSwtch_D_Stat,WiprFront_D_Stat
  wires:
  in_port/1 -> bus_selector/1  "Steering_Data_FD1_Ox83"
  bus_selector/1 -> AccButtnGapDecPress/1  "<AccButtnGapDecPress>"
  bus_selector/2 -> AccButtnGapIncPress/1  "<AccButtnGapIncPress>"
  bus_selector/3 -> AccButtnGapTogglePress/1  "<AccButtnGapTogglePress>"
  bus_selector/4 -> AhbStat_B_Dsply/1  "<AhbStat_B_Dsply>"
  bus_selector/5 -> AslButtnOnOffCnclPress/1  "<AslButtnOnOffCnclPress>"
  bus_selector/6 -> AslButtnOnOffPress/1  "<AslButtnOnOffPress>"
  bus_selector/7 -> CcAslButtnCnclPress/1  "<CcAslButtnCnclPress>"
  bus_selector/8 -> CcAslButtnCnclResPress/1  "<CcAslButtnCnclResPress>"
  bus_selector/9 -> CcAslButtnDeny_B_Actl/1  "<CcAslButtnDeny_B_Actl>"
  bus_selector/10 -> CcAslButtnIndxDecPress/1  "<CcAslButtnIndxDecPress>"
  bus_selector/11 -> CcAslButtnIndxIncPress/1  "<CcAslButtnIndxIncPress>"
  bus_selector/12 -> CcAslButtnOffCnclPress/1  "<CcAslButtnOffCnclPress>"
  bus_selector/13 -> CcAslButtnOnOffCncl/1  "<CcAslButtnOnOffCncl>"
  bus_selector/14 -> CcAslButtnOnPress/1  "<CcAslButtnOnPress>"
  bus_selector/15 -> CcAslButtnResDecPress/1  "<CcAslButtnResDecPress>"
  bus_selector/16 -> CcAslButtnResIncPress/1  "<CcAslButtnResIncPress>"
  bus_selector/17 -> CcAslButtnSetDecPress/1  "<CcAslButtnSetDecPress>"
  bus_selector/18 -> CcAslButtnSetIncPress/1  "<CcAslButtnSetIncPress>"
  bus_selector/19 -> CcAslButtnSetPress/1  "<CcAslButtnSetPress>"
  bus_selector/20 -> CcAsllButtnResPress/1  "<CcAsllButtnResPress>"
  bus_selector/21 -> CcButtnOffPress/1  "<CcButtnOffPress>"
  bus_selector/22 -> CcButtnOnOffCnclPress/1  "<CcButtnOnOffCnclPress>"
  bus_selector/23 -> CcButtnOnOffPress/1  "<CcButtnOnOffPress>"
  bus_selector/24 -> CcButtnOnPress/1  "<CcButtnOnPress>"
  bus_selector/25 -> HeadLghtHiCtrl_D_RqAhb/1  "<HeadLghtHiCtrl_D_RqAhb>"
  bus_selector/26 -> HeadLghtHiFlash_D_Actl/1  "<HeadLghtHiFlash_D_Actl>"
  bus_selector/27 -> HeadLghtHiFlash_D_Stat/1  "<HeadLghtHiFlash_D_Stat>"
  bus_selector/28 -> HeadLghtHiOn_B_StatAhb/1  "<HeadLghtHiOn_B_StatAhb>"
  bus_selector/29 -> LaSwtchPos_D_Stat/1  "<LaSwtchPos_D_Stat>"
  bus_selector/30 -> LghtAmb_D_Sns/1  "<LghtAmb_D_Sns>"
  bus_selector/31 -> TjaButtnOnOffPress/1  "<TjaButtnOnOffPress>"
  bus_selector/32 -> TurnLghtSwtch_D_Stat/1  "<TurnLghtSwtch_D_Stat>"
  bus_selector/33 -> WiprFrontSwtch_D_Stat/1  "<WiprFrontSwtch_D_Stat>"
  bus_selector/34 -> WiprFront_D_Stat/1  "<WiprFront_D_Stat>"

== system test_mdl_NI/Subsystem/GWM/Steering_Wheel_Data2_FD1_Ox81 ==
  in_port : Inport
  SelDrvMdeDec_B_RqDrv : Terminator
  SelDrvMdeInc_B_RqDrv : Terminator
  SelDrvMdeSwtch_D_Stat4 : Terminator
  SteEffortInc_B_RqDrv : Terminator
  SteWhlSwtchBack_B_Stat : Terminator
  SteWhlSwtchDown_B_Stat : Terminator
  SteWhlSwtchHome_B_Stat : Terminator
  SteWhlSwtchHud_B_Stat : Terminator
  SteWhlSwtchInfo_B_Stat : Terminator
  SteWhlSwtchIod_B_Stat : Terminator
  SteWhlSwtchLeft_B_Stat : Terminator
  SteWhlSwtchMed_B_Stat : Terminator
  SteWhlSwtchMenu_B_Stat : Terminator
  SteWhlSwtchNav_B_Stat : Terminator
  SteWhlSwtchOk_B_Stat : Terminator
  SteWhlSwtchPhon_B_Stat : Terminator
  SteWhlSwtchRght_B_Stat : Terminator
  SteWhlSwtchSet_B_Stat : Terminator
  SteWhlSwtchUp_B_Stat : Terminator
  SteWhlSwtchView_B_Stat : Terminator
  SuspDampInc_B_RqDrv : Terminator
  bus_selector : BusSelector  OutputSignals=SelDrvMdeDec_B_RqDrv,SelDrvMdeInc_B_RqDrv,SelDrvMdeSwtch_D_Stat4,SteEffortInc_B_RqDrv,SteWhlSwtchBack_B_Stat,SteWhlSwtchDown_B_Stat,SteWhlSwtchHome_B_Stat,SteWhlSwtchHud_B_Stat,SteWhlSwtchInfo_B_Stat,SteWhlSwtchIod_B_Stat,SteWhlSwtchLeft_B_Stat,SteWhlSwtchMed_B_Stat,SteWhlSwtchMenu_B_Stat,SteWhlSwtchNav_B_Stat,SteWhlSwtchOk_B_Stat,SteWhlSwtchPhon_B_Stat,SteWhlSwtchRght_B_Stat,SteWhlSwtchSet_B_Stat,SteWhlSwtchUp_B_Stat,SteWhlSwtchView_B_Stat,SuspDampInc_B_RqDrv
  wires:
  in_port/1 -> bus_selector/1  "Steering_Wheel_Data2_FD1_Ox81"
  bus_selector/1 -> SelDrvMdeDec_B_RqDrv/1  "<SelDrvMdeDec_B_RqDrv>"
  bus_selector/2 -> SelDrvMdeInc_B_RqDrv/1  "<SelDrvMdeInc_B_RqDrv>"
  bus_selector/3 -> SelDrvMdeSwtch_D_Stat4/1  "<SelDrvMdeSwtch_D_Stat4>"
  bus_selector/4 -> SteEffortInc_B_RqDrv/1  "<SteEffortInc_B_RqDrv>"
  bus_selector/5 -> SteWhlSwtchBack_B_Stat/1  "<SteWhlSwtchBack_B_Stat>"
  bus_selector/6 -> SteWhlSwtchDown_B_Stat/1  "<SteWhlSwtchDown_B_Stat>"
  bus_selector/7 -> SteWhlSwtchHome_B_Stat/1  "<SteWhlSwtchHome_B_Stat>"
  bus_selector/8 -> SteWhlSwtchHud_B_Stat/1  "<SteWhlSwtchHud_B_Stat>"
  bus_selector/9 -> SteWhlSwtchInfo_B_Stat/1  "<SteWhlSwtchInfo_B_Stat>"
  bus_selector/10 -> SteWhlSwtchIod_B_Stat/1  "<SteWhlSwtchIod_B_Stat>"
  bus_selector/11 -> SteWhlSwtchLeft_B_Stat/1  "<SteWhlSwtchLeft_B_Stat>"
  bus_selector/12 -> SteWhlSwtchMed_B_Stat/1  "<SteWhlSwtchMed_B_Stat>"
  bus_selector/13 -> SteWhlSwtchMenu_B_Stat/1  "<SteWhlSwtchMenu_B_Stat>"
  bus_selector/14 -> SteWhlSwtchNav_B_Stat/1  "<SteWhlSwtchNav_B_Stat>"
  bus_selector/15 -> SteWhlSwtchOk_B_Stat/1  "<SteWhlSwtchOk_B_Stat>"
  bus_selector/16 -> SteWhlSwtchPhon_B_Stat/1  "<SteWhlSwtchPhon_B_Stat>"
  bus_selector/17 -> SteWhlSwtchRght_B_Stat/1  "<SteWhlSwtchRght_B_Stat>"
  bus_selector/18 -> SteWhlSwtchSet_B_Stat/1  "<SteWhlSwtchSet_B_Stat>"
  bus_selector/19 -> SteWhlSwtchUp_B_Stat/1  "<SteWhlSwtchUp_B_Stat>"
  bus_selector/20 -> SteWhlSwtchView_B_Stat/1  "<SteWhlSwtchView_B_Stat>"
  bus_selector/21 -> SuspDampInc_B_RqDrv/1  "<SuspDampInc_B_RqDrv>"

== system test_mdl_NI/Subsystem/GWM/TCU_Send_Signals_FD1_Ox28B ==
  in_port : Inport
  EmgcyCallMute_D_Stat : Terminator
  OfbChrgSetSync_D_Rq : Terminator
  TelematicsSrvc_D_St : Terminator
  bus_selector : BusSelector  OutputSignals=EmgcyCallMute_D_Stat,OfbChrgSetSync_D_Rq,TelematicsSrvc_D_St
  wires:
  in_port/1 -> bus_selector/1  "TCU_Send_Signals_FD1_Ox28B"
  bus_selector/1 -> EmgcyCallMute_D_Stat/1  "<EmgcyCallMute_D_Stat>"
  bus_selector/2 -> OfbChrgSetSync_D_Rq/1  "<OfbChrgSetSync_D_Rq>"
  bus_selector/3 -> TelematicsSrvc_D_St/1  "<TelematicsSrvc_D_St>"

== system test_mdl_NI/Subsystem/GWM/TesterPhysicalReqVDM_FD1_Ox721 ==
  in_port : Inport
  TesterPhysicalReqVDM : Terminator
  bus_selector : BusSelector  OutputSignals=TesterPhysicalReqVDM
  wires:
  in_port/1 -> bus_selector/1  "TesterPhysicalReqVDM_FD1_Ox721"
  bus_selector/1 -> TesterPhysicalReqVDM/1  "<TesterPhysicalReqVDM>"

== system test_mdl_NI/Subsystem/GWM/TesterPhysicalResGWM_FD1_Ox71E ==
  in_port : Inport
  TesterPhysicalResGWM_F1 : Terminator
  bus_selector : BusSelector  OutputSignals=TesterPhysicalResGWM_F1
  wires:
  in_port/1 -> bus_selector/1  "TesterPhysicalResGWM_FD1_Ox71E"
  bus_selector/1 -> TesterPhysicalResGWM_F1/1  "<TesterPhysicalResGWM_F1>"

== system test_mdl_NI/Subsystem/GWM/Tire_Pressure_Data_FD1_Ox3B5 ==
  in_port : Inport
  Tire_Press_LF_Data : Terminator
  Tire_Press_LR_OLR_Data : Terminator
  Tire_Press_RF_Data : Terminator
  Tire_Press_RR_ORR_Data : Terminator
  bus_selector : BusSelector  OutputSignals=Tire_Press_LF_Data,Tire_Press_LR_OLR_Data,Tire_Press_RF_Data,Tire_Press_RR_ORR_Data
  wires:
  in_port/1 -> bus_selector/1  "Tire_Pressure_Data_FD1_Ox3B5"
  bus_selector/1 -> Tire_Press_LF_Data/1  "<Tire_Press_LF_Data>"
  bus_selector/2 -> Tire_Press_LR_OLR_Data/1  "<Tire_Press_LR_OLR_Data>"
  bus_selector/3 -> Tire_Press_RF_Data/1  "<Tire_Press_RF_Data>"
  bus_selector/4 -> Tire_Press_RR_ORR_Data/1  "<Tire_Press_RR_ORR_Data>"

== system test_mdl_NI/Subsystem/GWM/TrailerAid_Data3_FD1_Ox45C ==
  in_port : Inport
  TrlrAidEnbl_D2_Rq : Terminator
  TrlrAidSetup_D2_Rq : Terminator
  TrlrAnOffstDir_D_Mem : Terminator
  TrlrAnOffst_An_Mem : Terminator
  TrlrAxleToBmpr_L_Actl : Terminator
  TrlrBallToBmpr_L_Actl : Terminator
  TrlrIdType_D_Stat : Terminator
  TrlrId_No_Actl : Terminator
  TrlrRvrseCancl_B_Rq : Terminator
  TrlrTrgtOffst_L_Actl : Terminator
  TrlrTrgtPtrnId_No_Mem : Terminator
  TrlrTrgtToBmpr_L_Actl : Terminator
  bus_selector : BusSelector  OutputSignals=TrlrAidEnbl_D2_Rq,TrlrAidSetup_D2_Rq,TrlrAnOffstDir_D_Mem,TrlrAnOffst_An_Mem,TrlrAxleToBmpr_L_Actl,TrlrBallToBmpr_L_Actl,TrlrIdType_D_Stat,TrlrId_No_Actl,TrlrRvrseCancl_B_Rq,TrlrTrgtOffst_L_Actl,TrlrTrgtPtrnId_No_Mem,TrlrTrgtToBmpr_L_Actl
  wires:
  in_port/1 -> bus_selector/1  "TrailerAid_Data3_FD1_Ox45C"
  bus_selector/1 -> TrlrAidEnbl_D2_Rq/1  "<TrlrAidEnbl_D2_Rq>"
  bus_selector/2 -> TrlrAidSetup_D2_Rq/1  "<TrlrAidSetup_D2_Rq>"
  bus_selector/3 -> TrlrAnOffstDir_D_Mem/1  "<TrlrAnOffstDir_D_Mem>"
  bus_selector/4 -> TrlrAnOffst_An_Mem/1  "<TrlrAnOffst_An_Mem>"
  bus_selector/5 -> TrlrAxleToBmpr_L_Actl/1  "<TrlrAxleToBmpr_L_Actl>"
  bus_selector/6 -> TrlrBallToBmpr_L_Actl/1  "<TrlrBallToBmpr_L_Actl>"
  bus_selector/7 -> TrlrIdType_D_Stat/1  "<TrlrIdType_D_Stat>"
  bus_selector/8 -> TrlrId_No_Actl/1  "<TrlrId_No_Actl>"
  bus_selector/9 -> TrlrRvrseCancl_B_Rq/1  "<TrlrRvrseCancl_B_Rq>"
  bus_selector/10 -> TrlrTrgtOffst_L_Actl/1  "<TrlrTrgtOffst_L_Actl>"
  bus_selector/11 -> TrlrTrgtPtrnId_No_Mem/1  "<TrlrTrgtPtrnId_No_Mem>"
  bus_selector/12 -> TrlrTrgtToBmpr_L_Actl/1  "<TrlrTrgtToBmpr_L_Actl>"

== system test_mdl_NI/Subsystem/GWM/TrailerAid_Data_FD1_Ox45A ==
  in_port : Inport
  TrailCtlSwtch_B_Stat2 : Terminator
  TrlBrkInitOut_D_Rq : Terminator
  bus_selector : BusSelector  OutputSignals=TrailCtlSwtch_B_Stat2,TrlBrkInitOut_D_Rq
  wires:
  in_port/1 -> bus_selector/1  "TrailerAid_Data_FD1_Ox45A"
  bus_selector/1 -> TrailCtlSwtch_B_Stat2/1  "<TrailCtlSwtch_B_Stat2>"
  bus_selector/2 -> TrlBrkInitOut_D_Rq/1  "<TrlBrkInitOut_D_Rq>"

== system test_mdl_NI/Subsystem/GWM/TrailerAid_Stat1_FD1_Ox452 ==
  in_port : Inport
  TrlrSnsId_No_Actl : Terminator
  bus_selector : BusSelector  OutputSignals=TrlrSnsId_No_Actl
  wires:
  in_port/1 -> bus_selector/1  "TrailerAid_Stat1_FD1_Ox452"
  bus_selector/1 -> TrlrSnsId_No_Actl/1  "<TrlrSnsId_No_Actl>"

== system test_mdl_NI/Subsystem/GWM/TrailerAid_Stat2_FD1_Ox457 ==
  in_port : Inport
  TrlrHitYaw_AnRate_Actl : Terminator
  TrlrHitchYaw_An_Actl : Terminator
  TrlrHitchYaw_D_Stat : Terminator
  TrlrYawWActl_D_Qf : Terminator
  TrlrYaw_W_Actl : Terminator
  bus_selector : BusSelector  OutputSignals=TrlrHitYaw_AnRate_Actl,TrlrHitchYaw_An_Actl,TrlrHitchYaw_D_Stat,TrlrYawWActl_D_Qf,TrlrYaw_W_Actl
  wires:
  in_port/1 -> bus_selector/1  "TrailerAid_Stat2_FD1_Ox457"
  bus_selector/1 -> TrlrHitYaw_AnRate_Actl/1  "<TrlrHitYaw_AnRate_Actl>"
  bus_selector/2 -> TrlrHitchYaw_An_Actl/1  "<TrlrHitchYaw_An_Actl>"
  bus_selector/3 -> TrlrHitchYaw_D_Stat/1  "<TrlrHitchYaw_D_Stat>"
  bus_selector/4 -> TrlrYawWActl_D_Qf/1  "<TrlrYawWActl_D_Qf>"
  bus_selector/5 -> TrlrYaw_W_Actl/1  "<TrlrYaw_W_Actl>"

== system test_mdl_NI/Subsystem/GWM/TrailerBrakeInfo_FD1_Ox445 ==
  in_port : Inport
  StopLamp_B_RqTrlrBrk : Terminator
  TrlBrkInitOut_D_Stat : Terminator
  TrlrBrkActCirct_B_Falt : Terminator
  TrlrBrkActCnnct_B_Actl : Terminator
  TrlrBrkCtl_B_Falt : Terminator
  TrlrBrkDcnnt_B_Actl : Terminator
  TrlrBrkDsply_B_Rq : Terminator
  TrlrBrkGain_No_Actl : Terminator
  TrlrBrkMde_D_Actl : Terminator
  TrlrBrkOut_No_Dsply : Terminator
  bus_selector : BusSelector  OutputSignals=StopLamp_B_RqTrlrBrk,TrlBrkInitOut_D_Stat,TrlrBrkActCirct_B_Falt,TrlrBrkActCnnct_B_Actl,TrlrBrkCtl_B_Falt,TrlrBrkDcnnt_B_Actl,TrlrBrkDsply_B_Rq,TrlrBrkGain_No_Actl,TrlrBrkMde_D_Actl,TrlrBrkOut_No_Dsply
  wires:
  in_port/1 -> bus_selector/1  "TrailerBrakeInfo_FD1_Ox445"
  bus_selector/1 -> StopLamp_B_RqTrlrBrk/1  "<StopLamp_B_RqTrlrBrk>"
  bus_selector/2 -> TrlBrkInitOut_D_Stat/1  "<TrlBrkInitOut_D_Stat>"
  bus_selector/3 -> TrlrBrkActCirct_B_Falt/1  "<TrlrBrkActCirct_B_Falt>"
  bus_selector/4 -> TrlrBrkActCnnct_B_Actl/1  "<TrlrBrkActCnnct_B_Actl>"
  bus_selector/5 -> TrlrBrkCtl_B_Falt/1  "<TrlrBrkCtl_B_Falt>"
  bus_selector/6 -> TrlrBrkDcnnt_B_Actl/1  "<TrlrBrkDcnnt_B_Actl>"
  bus_selector/7 -> TrlrBrkDsply_B_Rq/1  "<TrlrBrkDsply_B_Rq>"
  bus_selector/8 -> TrlrBrkGain_No_Actl/1  "<TrlrBrkGain_No_Actl>"
  bus_selector/9 -> TrlrBrkMde_D_Actl/1  "<TrlrBrkMde_D_Actl>"
  bus_selector/10 -> TrlrBrkOut_No_Dsply/1  "<TrlrBrkOut_No_Dsply>"

== system test_mdl_NI/Subsystem/GWM/TrailerInfo_2_FD1_Ox47A ==
  in_port : Inport
  TrlrAidCtl_U_RqDrv : Terminator
  TrlrAidSwtch_D_RqDrv : Terminator
  bus_selector : BusSelector  OutputSignals=TrlrAidCtl_U_RqDrv,TrlrAidSwtch_D_RqDrv
  wires:
  in_port/1 -> bus_selector/1  "TrailerInfo_2_FD1_Ox47A"
  bus_selector/1 -> TrlrAidCtl_U_RqDrv/1  "<TrlrAidCtl_U_RqDrv>"
  bus_selector/2 -> TrlrAidSwtch_D_RqDrv/1  "<TrlrAidSwtch_D_RqDrv>"

== system test_mdl_NI/Subsystem/GWM/TrailerInfo_FD1_Ox443 ==
  in_port : Inport
  ParkLampTrlrOut_B_Stat : Terminator
  StopLampTrlrOut_B_Stat : Terminator
  TrlrBattChrg_D_Stat : Terminator
  TrlrLampCnnct_B_Actl : Terminator
  TrlrLampCtl_D_Stat : Terminator
  TurnLampTrlrRl_B_Stat : Terminator
  TurnLampTrlrRr_B_Stat : Terminator
  bus_selector : BusSelector  OutputSignals=ParkLampTrlrOut_B_Stat,StopLampTrlrOut_B_Stat,TrlrBattChrg_D_Stat,TrlrLampCnnct_B_Actl,TrlrLampCtl_D_Stat,TurnLampTrlrRl_B_Stat,TurnLampTrlrRr_B_Stat
  wires:
  in_port/1 -> bus_selector/1  "TrailerInfo_FD1_Ox443"
  bus_selector/1 -> ParkLampTrlrOut_B_Stat/1  "<ParkLampTrlrOut_B_Stat>"
  bus_selector/2 -> StopLampTrlrOut_B_Stat/1  "<StopLampTrlrOut_B_Stat>"
  bus_selector/3 -> TrlrBattChrg_D_Stat/1  "<TrlrBattChrg_D_Stat>"
  bus_selector/4 -> TrlrLampCnnct_B_Actl/1  "<TrlrLampCnnct_B_Actl>"
  bus_selector/5 -> TrlrLampCtl_D_Stat/1  "<TrlrLampCtl_D_Stat>"
  bus_selector/6 -> TurnLampTrlrRl_B_Stat/1  "<TurnLampTrlrRl_B_Stat>"
  bus_selector/7 -> TurnLampTrlrRr_B_Stat/1  "<TurnLampTrlrRr_B_Stat>"

== system test_mdl_NI/Subsystem/GWM/Voltage_Power_Data2_FD1_Ox45F ==
  in_port : Inport
  CoolFanDcdc_D_Rq : Terminator
  DcdcClntFlw_D_Rq : Terminator
  bus_selector : BusSelector  OutputSignals=CoolFanDcdc_D_Rq,DcdcClntFlw_D_Rq
  wires:
  in_port/1 -> bus_selector/1  "Voltage_Power_Data2_FD1_Ox45F"
  bus_selector/1 -> CoolFanDcdc_D_Rq/1  "<CoolFanDcdc_D_Rq>"
  bus_selector/2 -> DcdcClntFlw_D_Rq/1  "<DcdcClntFlw_D_Rq>"

== system test_mdl_NI/Subsystem/GWM/Yaw_Data_FD1_Ox91 ==
  in_port : Inport
  VehRolWActl_D_Qf : Terminator
  VehRol_W_Actl : Terminator
  VehRollYawW_No_Cs : Terminator
  VehRollYaw_No_Cnt : Terminator
  VehYawWActl_D_Qf : Terminator
  VehYaw_W_Actl : Terminator
  bus_selector : BusSelector  OutputSignals=VehRolWActl_D_Qf,VehRol_W_Actl,VehRollYawW_No_Cs,VehRollYaw_No_Cnt,VehYawWActl_D_Qf,VehYaw_W_Actl
  wires:
  in_port/1 -> bus_selector/1  "Yaw_Data_FD1_Ox91"
  bus_selector/1 -> VehRolWActl_D_Qf/1  "<VehRolWActl_D_Qf>"
  bus_selector/2 -> VehRol_W_Actl/1  "<VehRol_W_Actl>"
  bus_selector/3 -> VehRollYawW_No_Cs/1  "<VehRollYawW_No_Cs>"
  bus_selector/4 -> VehRollYaw_No_Cnt/1  "<VehRollYaw_No_Cnt>"
  bus_selector/5 -> VehYawWActl_D_Qf/1  "<VehYawWActl_D_Qf>"
  bus_selector/6 -> VehYaw_W_Actl/1  "<VehYaw_W_Actl>"

== system test_mdl_NI/Subsystem/IPMA_ADAS/ACCDATA_2_Ox187 ==
  in_port : Inport
  CmbbBaSens_D_Rq : Terminator
  CmbbBrkDecel_A_Rq : Terminator
  CmbbBrkDecel_B_Rq : Terminator
  CmbbBrkDecel_No_Cnt : Terminator
  CmbbBrkDecel_No_Cs : Terminator
  CmbbBrkPrchg_D_Rq : Terminator
  HudBlk1_B_Rq : Terminator
  HudBlk2_B_Rq : Terminator
  HudBlk3_B_Rq : Terminator
  HudDsplyIntns_No_Actl : Terminator
  HudFlashRate_D_Actl : Terminator
  bus_selector : BusSelector  OutputSignals=CmbbBaSens_D_Rq,CmbbBrkDecel_A_Rq,CmbbBrkDecel_B_Rq,CmbbBrkDecel_No_Cnt,CmbbBrkDecel_No_Cs,CmbbBrkPrchg_D_Rq,HudBlk1_B_Rq,HudBlk2_B_Rq,HudBlk3_B_Rq,HudDsplyIntns_No_Actl,HudFlashRate_D_Actl
  wires:
  in_port/1 -> bus_selector/1  "ACCDATA_2_Ox187"
  bus_selector/1 -> CmbbBaSens_D_Rq/1  "<CmbbBaSens_D_Rq>"
  bus_selector/2 -> CmbbBrkDecel_A_Rq/1  "<CmbbBrkDecel_A_Rq>"
  bus_selector/3 -> CmbbBrkDecel_B_Rq/1  "<CmbbBrkDecel_B_Rq>"
  bus_selector/4 -> CmbbBrkDecel_No_Cnt/1  "<CmbbBrkDecel_No_Cnt>"
  bus_selector/5 -> CmbbBrkDecel_No_Cs/1  "<CmbbBrkDecel_No_Cs>"
  bus_selector/6 -> CmbbBrkPrchg_D_Rq/1  "<CmbbBrkPrchg_D_Rq>"
  bus_selector/7 -> HudBlk1_B_Rq/1  "<HudBlk1_B_Rq>"
  bus_selector/8 -> HudBlk2_B_Rq/1  "<HudBlk2_B_Rq>"
  bus_selector/9 -> HudBlk3_B_Rq/1  "<HudBlk3_B_Rq>"
  bus_selector/10 -> HudDsplyIntns_No_Actl/1  "<HudDsplyIntns_No_Actl>"
  bus_selector/11 -> HudFlashRate_D_Actl/1  "<HudFlashRate_D_Actl>"

== system test_mdl_NI/Subsystem/IPMA_ADAS/ACCDATA_3_Ox18A ==
  in_port : Inport
  AccFllwMde_B_Dsply : Terminator
  AccMemEnbl_B_RqDrv : Terminator
  AccMsgTxt_D2_Rq : Terminator
  AccStopMde_B_Dsply : Terminator
  AccStopRes_B_Dsply : Terminator
  AccStopStat_D_Dsply : Terminator
  AccTGap_B_Dsply : Terminator
  AccTGap_D_Dsply : Terminator
  AccTrgDist2_D_Dsply : Terminator
  AccWarn_D_Dsply : Terminator
  CadsAlignIncplt_B_Actl : Terminator
  CadsRadrBlck_B_Actl : Terminator
  CmbbPostEvnt_B_Dsply : Terminator
  FcwAudioWarn_B_Rq : Terminator
  FcwDeny_B_Dsply : Terminator
  FcwMemSens_D_Actl : Terminator
  FcwMemStat_B_Actl : Terminator
  FcwMsgTxt_D_Rq : Terminator
  FcwVisblWarn_B_Rq : Terminator
  FdaMem_B_Stat : Terminator
  HaDsply_No_Cnt : Terminator
  HaDsply_No_Cs : Terminator
  IaccLamp_D_Rq : Terminator
  TjaMsgTxt_D_Dsply : Terminator
  TjaWarn_D_Rq : Terminator
  Tja_D_Stat : Terminator
  bus_selector : BusSelector  OutputSignals=AccFllwMde_B_Dsply,AccMemEnbl_B_RqDrv,AccMsgTxt_D2_Rq,AccStopMde_B_Dsply,AccStopRes_B_Dsply,AccStopStat_D_Dsply,AccTGap_B_Dsply,AccTGap_D_Dsply,AccTrgDist2_D_Dsply,AccWarn_D_Dsply,CadsAlignIncplt_B_Actl,CadsRadrBlck_B_Actl,CmbbPostEvnt_B_Dsply,FcwAudioWarn_B_Rq,FcwDeny_B_Dsply,FcwMemSens_D_Actl,FcwMemStat_B_Actl,FcwMsgTxt_D_Rq,FcwVisblWarn_B_Rq,FdaMem_B_Stat,HaDsply_No_Cnt,HaDsply_No_Cs,IaccLamp_D_Rq,TjaMsgTxt_D_Dsply,TjaWarn_D_Rq,Tja_D_Stat
  wires:
  in_port/1 -> bus_selector/1  "ACCDATA_3_Ox18A"
  bus_selector/1 -> AccFllwMde_B_Dsply/1  "<AccFllwMde_B_Dsply>"
  bus_selector/2 -> AccMemEnbl_B_RqDrv/1  "<AccMemEnbl_B_RqDrv>"
  bus_selector/3 -> AccMsgTxt_D2_Rq/1  "<AccMsgTxt_D2_Rq>"
  bus_selector/4 -> AccStopMde_B_Dsply/1  "<AccStopMde_B_Dsply>"
  bus_selector/5 -> AccStopRes_B_Dsply/1  "<AccStopRes_B_Dsply>"
  bus_selector/6 -> AccStopStat_D_Dsply/1  "<AccStopStat_D_Dsply>"
  bus_selector/7 -> AccTGap_B_Dsply/1  "<AccTGap_B_Dsply>"
  bus_selector/8 -> AccTGap_D_Dsply/1  "<AccTGap_D_Dsply>"
  bus_selector/9 -> AccTrgDist2_D_Dsply/1  "<AccTrgDist2_D_Dsply>"
  bus_selector/10 -> AccWarn_D_Dsply/1  "<AccWarn_D_Dsply>"
  bus_selector/11 -> CadsAlignIncplt_B_Actl/1  "<CadsAlignIncplt_B_Actl>"
  bus_selector/12 -> CadsRadrBlck_B_Actl/1  "<CadsRadrBlck_B_Actl>"
  bus_selector/13 -> CmbbPostEvnt_B_Dsply/1  "<CmbbPostEvnt_B_Dsply>"
  bus_selector/14 -> FcwAudioWarn_B_Rq/1  "<FcwAudioWarn_B_Rq>"
  bus_selector/15 -> FcwDeny_B_Dsply/1  "<FcwDeny_B_Dsply>"
  bus_selector/16 -> FcwMemSens_D_Actl/1  "<FcwMemSens_D_Actl>"
  bus_selector/17 -> FcwMemStat_B_Actl/1  "<FcwMemStat_B_Actl>"
  bus_selector/18 -> FcwMsgTxt_D_Rq/1  "<FcwMsgTxt_D_Rq>"
  bus_selector/19 -> FcwVisblWarn_B_Rq/1  "<FcwVisblWarn_B_Rq>"
  bus_selector/20 -> FdaMem_B_Stat/1  "<FdaMem_B_Stat>"
  bus_selector/21 -> HaDsply_No_Cnt/1  "<HaDsply_No_Cnt>"
  bus_selector/22 -> HaDsply_No_Cs/1  "<HaDsply_No_Cs>"
  bus_selector/23 -> IaccLamp_D_Rq/1  "<IaccLamp_D_Rq>"
  bus_selector/24 -> TjaMsgTxt_D_Dsply/1  "<TjaMsgTxt_D_Dsply>"
  bus_selector/25 -> TjaWarn_D_Rq/1  "<TjaWarn_D_Rq>"
  bus_selector/26 -> Tja_D_Stat/1  "<Tja_D_Stat>"

== system test_mdl_NI/Subsystem/IPMA_ADAS/ACCDATA_Ox186 ==
  in_port : Inport
  AccAutoResum_D_Rq : Terminator
  AccBrkDecel_B_Rq : Terminator
  AccBrkPrchg_B_Rq : Terminator
  AccBrkPrkEl_B_Rq : Terminator
  AccBrkPulse_B_Rq : Terminator
  AccBrkTot_A_Rq : Terminator
  AccCancl_B_Rq : Terminator
  AccDeny_B_Rq : Terminator
  AccPrpl_A_Pred : Terminator
  AccPrpl_A_Rq : Terminator
  AccResumEnbl_B_Rq : Terminator
  AccStopStat_B_Rq : Terminator
  AccVeh_V_Trg : Terminator
  CmbbDeny_B_Actl : Terminator
  CmbbEngTqMn_B_Rq : Terminator
  CmbbOvrrd_B_RqDrv : Terminator
  Cmbb_B_Enbl : Terminator
  bus_selector : BusSelector  OutputSignals=AccAutoResum_D_Rq,AccBrkDecel_B_Rq,AccBrkPrchg_B_Rq,AccBrkPrkEl_B_Rq,AccBrkPulse_B_Rq,AccBrkTot_A_Rq,AccCancl_B_Rq,AccDeny_B_Rq,AccPrpl_A_Pred,AccPrpl_A_Rq,AccResumEnbl_B_Rq,AccStopStat_B_Rq,AccVeh_V_Trg,CmbbDeny_B_Actl,CmbbEngTqMn_B_Rq,CmbbOvrrd_B_RqDrv,Cmbb_B_Enbl
  wires:
  in_port/1 -> bus_selector/1  "ACCDATA_Ox186"
  bus_selector/1 -> AccAutoResum_D_Rq/1  "<AccAutoResum_D_Rq>"
  bus_selector/2 -> AccBrkDecel_B_Rq/1  "<AccBrkDecel_B_Rq>"
  bus_selector/3 -> AccBrkPrchg_B_Rq/1  "<AccBrkPrchg_B_Rq>"
  bus_selector/4 -> AccBrkPrkEl_B_Rq/1  "<AccBrkPrkEl_B_Rq>"
  bus_selector/5 -> AccBrkPulse_B_Rq/1  "<AccBrkPulse_B_Rq>"
  bus_selector/6 -> AccBrkTot_A_Rq/1  "<AccBrkTot_A_Rq>"
  bus_selector/7 -> AccCancl_B_Rq/1  "<AccCancl_B_Rq>"
  bus_selector/8 -> AccDeny_B_Rq/1  "<AccDeny_B_Rq>"
  bus_selector/9 -> AccPrpl_A_Pred/1  "<AccPrpl_A_Pred>"
  bus_selector/10 -> AccPrpl_A_Rq/1  "<AccPrpl_A_Rq>"
  bus_selector/11 -> AccResumEnbl_B_Rq/1  "<AccResumEnbl_B_Rq>"
  bus_selector/12 -> AccStopStat_B_Rq/1  "<AccStopStat_B_Rq>"
  bus_selector/13 -> AccVeh_V_Trg/1  "<AccVeh_V_Trg>"
  bus_selector/14 -> CmbbDeny_B_Actl/1  "<CmbbDeny_B_Actl>"
  bus_selector/15 -> CmbbEngTqMn_B_Rq/1  "<CmbbEngTqMn_B_Rq>"
  bus_selector/16 -> CmbbOvrrd_B_RqDrv/1  "<CmbbOvrrd_B_RqDrv>"
  bus_selector/17 -> Cmbb_B_Enbl/1  "<Cmbb_B_Enbl>"

== system test_mdl_NI/Subsystem/IPMA_ADAS/AutoDriveBeam_Data1_Ox3D4 ==
  in_port : Inport
  AdbBrdr1CritLeft_T_Stat : Terminator
  AdbBrdr1CritRigh_T_Stat : Terminator
  AdbBrdr1DistLeft_D_Stat : Terminator
  AdbBrdr1DistRigh_D_Stat : Terminator
  AdbBrdr1Left_An_Rq : Terminator
  AdbBrdr1Low_An_Rq : Terminator
  AdbBrdr1Right_An_Rq : Terminator
  AdbBrdr1Up_An_Rq : Terminator
  AdbIntns1_D_Rq : Terminator
  AdbMde1_D_Rq : Terminator
  bus_selector : BusSelector  OutputSignals=AdbBrdr1CritLeft_T_Stat,AdbBrdr1CritRigh_T_Stat,AdbBrdr1DistLeft_D_Stat,AdbBrdr1DistRigh_D_Stat,AdbBrdr1Left_An_Rq,AdbBrdr1Low_An_Rq,AdbBrdr1Right_An_Rq,AdbBrdr1Up_An_Rq,AdbIntns1_D_Rq,AdbMde1_D_Rq
  wires:
  in_port/1 -> bus_selector/1  "AutoDriveBeam_Data1_Ox3D4"
  bus_selector/1 -> AdbBrdr1CritLeft_T_Stat/1  "<AdbBrdr1CritLeft_T_Stat>"
  bus_selector/2 -> AdbBrdr1CritRigh_T_Stat/1  "<AdbBrdr1CritRigh_T_Stat>"
  bus_selector/3 -> AdbBrdr1DistLeft_D_Stat/1  "<AdbBrdr1DistLeft_D_Stat>"
  bus_selector/4 -> AdbBrdr1DistRigh_D_Stat/1  "<AdbBrdr1DistRigh_D_Stat>"
  bus_selector/5 -> AdbBrdr1Left_An_Rq/1  "<AdbBrdr1Left_An_Rq>"
  bus_selector/6 -> AdbBrdr1Low_An_Rq/1  "<AdbBrdr1Low_An_Rq>"
  bus_selector/7 -> AdbBrdr1Right_An_Rq/1  "<AdbBrdr1Right_An_Rq>"
  bus_selector/8 -> AdbBrdr1Up_An_Rq/1  "<AdbBrdr1Up_An_Rq>"
  bus_selector/9 -> AdbIntns1_D_Rq/1  "<AdbIntns1_D_Rq>"
  bus_selector/10 -> AdbMde1_D_Rq/1  "<AdbMde1_D_Rq>"
